simulink model "Aloe_E_Cell_Project_2016"  (R2016b)
settings: Solver=VariableStepAuto  StartTime=0.0  StopTime=0.14  RelTol=1e-3
undefined symbols (not defined in the file): D1, Delta
libraries: powerlib x218, powerlib_meascontrol x6, simulink x2
(part 1 of 2)
settings Model: Creator=mdeat  LastModifiedBy=mdeat
settings DataIOCC: ReturnWorkspaceOutputs=on
settings SFSimCC: SimUseLocalCustomCode=on
settings RTWCC: RTWUseLocalCustomCode=on

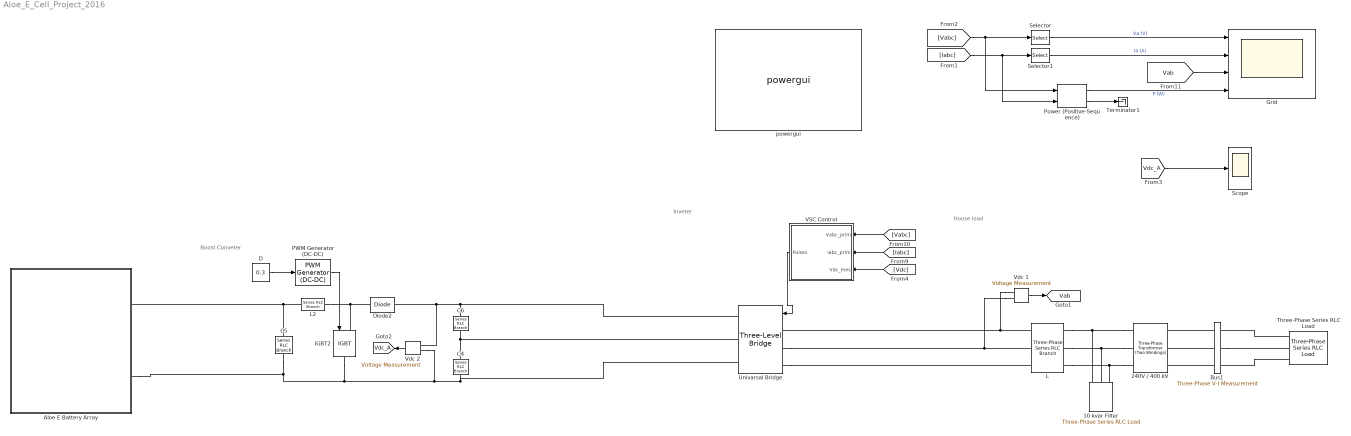
== system Aloe_E_Cell_Project_2016 ==
  note: Boost Conveter
  note: House load
  note: Inveter
  10 kvar Filter : powerlib/Elements/Three-Phase Series RLC Load  LConnTagsString=A|B|C  Configuration=Y (grounded)  NominalVoltage=240  Vabc=[1e3 1e3 1e3]  Vabcp=[1e3 1e3 1e3]  NominalFrequency=50  UnbalancedPower=off  ActivePower=100  InductivePower=0  CapacitivePower=10e3  Pabc=[10e3 9e3 11e3]  QLabc=[100 90 110]  QCabc=[100 90 110]  Pabcp=[10e3 9e3 11e3]  QLabcp=[100 90 110]  QCabcp=[100 90 110]  Measurements=None  LoadType=constant Z
  240V / 400 kV : powerlib/Elements/Three-Phase Transformer (Two Windings)  Winding1Connection=Yg  Winding2Connection=Delta (D1)  CoreType=Three single-phase transformers  SetSaturation=off  Hysteresis=off  DataFile='hysteresis'  SetInitialFlux=off  Measurements=None  UNITS=pu  NominalPower=[100 , 50 ]  Winding1=[ 400 , 0.001 , 0.03 ]  Winding2=[ 260 , 0.001 , 0.03 ]  Rm=500  Lm=500  L0=0.5  Saturation=[ 0,0 ; 0.0024,1.2 ; 1.0,1.52 ]  InitialFluxes=[ 0.8 , -0.8 , 0.7 ]  BreakLoop=off  DiscreteSolver=Trapezoidal iterative  DataType=off  TransfoNumber=0
  Aloe E Battery Array : Subsystem
      mask Display: image('$imagefile'); % Use "Edit Image" on toolstrip to change.
  Bus1 : powerlib/Measurements/Three-Phase V-I Measurement  VoltageMeasurement=phase-to-ground  SetLabelV=on  LabelV=Vabc  Vpu=off  VpuLL=off  CurrentMeasurement=yes  SetLabelI=on  LabelI=Iabc  Ipu=off  Pbase=100e6  Vbase=500e3  OutputType=Magnitude  PhasorSimulation=off  PSBequivalent=0
  C4 : powerlib/Elements/Series RLC Branch  LConnTagsString=__new0  RConnTagsString=__new0  BranchType=C  Resistance=1.0  Inductance=1.0  SetiL0=off  InitialCurrent=0  Capacitance=2e-4  Setx0=off  InitialVoltage=0  Measurements=None
  C5 : powerlib/Elements/Series RLC Branch  LConnTagsString=__new0  RConnTagsString=__new0  BranchType=C  Resistance=1.0  Inductance=1.0  SetiL0=off  InitialCurrent=0  Capacitance=100e-6  Setx0=off  InitialVoltage=0  Measurements=Branch voltage
  C6 : powerlib/Elements/Series RLC Branch  LConnTagsString=__new0  RConnTagsString=__new0  BranchType=C  Resistance=1.0  Inductance=1.0  SetiL0=off  InitialCurrent=0  Capacitance=12e-03  Setx0=off  InitialVoltage=0  Measurements=None
  D : Constant  Value=0.3
  Diode2 : powerlib/Power Electronics/Diode  Ron=1e-4  Lon=0  Vf=0  IC=0  UseSnubber=off  Rs=inf  Cs=inf  Measurements=off
  Grid : Scope  NumInputPorts=4
  IGBT2 : powerlib/Power Electronics/IGBT  Ron=0.001  Lon=0  Vf=0  Tf=0  Tt=0  IC=0  Rs=1e5  Cs=inf  Measurements=off
  L : powerlib/Elements/Three-Phase Series RLC Branch  LConnTagsString=A|B|C  RConnTagsString=A|B|C  BranchType=RL  Resistance=500e-6*377/50/2  Inductance=500e-6/2  Capacitance=inf  Measurements=None
  L2 : powerlib/Elements/Series RLC Branch  LConnTagsString=__new0  RConnTagsString=__new0  BranchType=RL  Resistance=0.005  Inductance=5e-3  SetiL0=off  InitialCurrent=0  Capacitance=1e-6  Setx0=off  InitialVoltage=0  Measurements=None
  PWM Generator (DC-DC) : powerlib_meascontrol/Pulse & Signal Generators/PWM Generator (DC-DC)  Fsw=20e3  Ts=0
  Power (Positive-Sequence) : powerlib_meascontrol/Measurements/Power (Positive-Sequence)  Freq=60  Vinit=[0, 0]  Iinit=[0, 0]  Ts=0.0001
  Scope : Scope
  Selector : Selector  InputPortWidth=3  IndexOptions=Index vector (dialog)  Indices=[1]  OutputSizes=1
  Selector1 : Selector  InputPortWidth=3  IndexOptions=Index vector (dialog)  Indices=[1]  OutputSizes=1
  Terminator1 : Terminator
  Three-Phase Series RLC Load : powerlib/Elements/Three-Phase Series RLC Load  LConnTagsString=A|B|C  Configuration=Y (grounded)  NominalVoltage=400  Vabc=[1e3 1e3 1e3]  Vabcp=[1e3 1e3 1e3]  NominalFrequency=50  UnbalancedPower=off  ActivePower=1000  InductivePower=0  CapacitivePower=100  Pabc=[10e3 9e3 11e3]  QLabc=[100 90 110]  QCabc=[100 90 110]  Pabcp=[10e3 9e3 11e3]  QLabcp=[100 90 110]  QCabcp=[100 90 110]  Measurements=None  LoadType=constant Z
  Univarsal Bridge : powerlib/Power Electronics/Three-Level Bridge  Arms=3  SnubberResistance=1e6  SbubberCapacitance=inf  Device=IGBT / Diodes  Ron=0.2e-3  ForwardVoltages="[  0  0 ]"  Measurements=None
  VSC Control : Subsystem  mask(VSC Main Controller){nom=[ 1000  50 ], Vnom=[ 2000 260 ], Vnom_dc=220, RLxfo=[0.002  0.06 ], RLchoke=[2e-3  250e-6  ], K_VDCreg=[7  800], K_Ireg=[0.3 20], Ts=0.0001}
      mask prompts: nom "Nominal power and frequency [ Pnom(VA)  Fnom(Hz) ]:"; Vnom "Nominal primary and secondary voltages (Vrms LL) [ Vnom_prim   Vnom_sec ]:"; Vnom_dc "Nominal DC bus voltage (V):"; RLxfo "Total transformer leakage impedance (pu/Pnom) [ Rxfo  Lxf ]"; RLchoke "Choke impedance [ R(ohm) L(H) ]"; K_VDCreg "VDC regultator gains [ Kp  Ki ]:"; K_Ireg "Current regulator gains [ Kp  Ki ]:"; Ts "Sample time"
      mask init:
      | Pnom=nom(1);
      | Fnom=nom(2);
      | Vnom_prim=Vnom(1);
      | Vnom_sec=Vnom(2);
      | Zbase=Vnom_sec^2/Pnom;
      | Rtot_pu=RLxfo(1) + RLchoke(1)/Zbase;
      | Ltot_pu=RLxfo(2) + RLchoke(2)/(Zbase/(2*pi*Fnom));
      | Kp_VDCreg=K_VDCreg(1);
      | Ki_VDCreg=K_VDCreg(2);
      | Kp_Ireg=K_Ireg(1);
      | Ki_Ireg=K_Ireg(2);
      | Vdc_ref=Vnom_dc;
      | % Used to determine initial value of Boost Control (MPPT)
      | assignin('base','Vdc_ref_Inv',Vdc_ref);
  Vdc 1 : powerlib/Measurements/Voltage Measurement  Tag=PoWeRsYsTeMmEaSuReMeNt  PhasorSimulation=off  OutputType=Magnitude  PSBequivalent=0
  Vdc 2 : powerlib/Measurements/Voltage Measurement  Tag=PoWeRsYsTeMmEaSuReMeNt  PhasorSimulation=off  OutputType=Magnitude  PSBequivalent=0
  powergui : powerlib/powergui  Priority=1  SimulationMode=Discrete  SampleTime=1e-5  frequency=60  Iterations=50  frequencyindice=0  Pbase=100e6  ErrMax=1e-4  UnitsV=kV  UnitsW=MW  buscounter=0  FunctionMessages=off  echomessages=off  EnableUseOfTLC=off  CurrentSourceSwitches=off  DisableSnubberDevices=off  DisableRonSwitches=off  DisableVfSwitches=off  DisplayEquations=off  AutomaticDiscreteSolvers=off  SolverType=Tustin/Backward Euler (TBE)  Interpol=off  ExternalGateDelay=off  methode=off  Ts=100  x0status=blocks  SPID=on  SwTol=0  HookPort=off  NonlinearTolerance=1e-4  nMaxIteration=100  ContinueOnMaxIteration=off  RestoreLinks=warning  ResistiveCurrentMeasurement=off  Frange=[0:2:500]  Ylog=off  Xlog=on  ShowGrid=off  save=off  variable=ZData  structure=0  ZoomFFT=off  StartTime=0.0  cycles=1  DisplayStyle=1  fundamental=60  FreqAxis=off  MaxFrequency=1000  frequencyindicesteady=1  RmsSteady=1  display=off
  tag scope: Vab=global, Vdc_A=global
  wires:
  Selector/1 -> Grid/1  "Va (V)"
  [Vab] -> Grid/3
  Selector1/1 -> Grid/2  "Ia (A)"
  [Vdc_A] -> Scope/1
  Power (Positive-Sequence)/1 -> Grid/4  "P (W)"
  Vdc 2/1 -> [Vdc_A]
  PWM Generator (DC-DC)/1 -> IGBT2/1
  D/1 -> PWM Generator (DC-DC)/1
  VSC Control/1(Pulses) -> Univarsal Bridge/1
  [Vabc] -> VSC Control/1(Vabc_prim)
  [Vdc] -> VSC Control/3(Vdc_mes)
  [Iabc] -> VSC Control/2(Iabc_prim)
  [Vabc] -> Power (Positive-Sequence)/1, Selector/1
  Power (Positive-Sequence)/2 -> Terminator1/1
  [Iabc] -> Power (Positive-Sequence)/2, Selector1/1
  Vdc 1/1 -> [Vab]
  connections:
  C5/LConn1 -- L2/LConn1 -- Aloe E Battery Array/RConn1
  Vdc 2/LConn2 -- Univarsal Bridge/RConn3 -- C4/RConn1 -- IGBT2/RConn1 -- C5/RConn1 -- Aloe E Battery Array/RConn2
  Diode2/RConn1 -- Univarsal Bridge/RConn1 -- C6/LConn1 -- Vdc 2/LConn1
  L2/RConn1 -- Diode2/LConn1 -- IGBT2/LConn1
  Vdc 1/LConn1 -- Univarsal Bridge/LConn1 -- L/LConn1
  240V / 400 kV/RConn3 -- L/RConn3 -- 10 kvar Filter/LConn3
  Vdc 1/LConn2 -- Univarsal Bridge/LConn2 -- L/LConn2
  240V / 400 kV/RConn1 -- L/RConn1 -- 10 kvar Filter/LConn1
  240V / 400 kV/RConn2 -- L/RConn2 -- 10 kvar Filter/LConn2
  Bus1/LConn3 -- 240V / 400 kV/LConn3
  Three-Phase Series RLC Load/LConn1 -- Bus1/RConn1
  Three-Phase Series RLC Load/LConn3 -- Bus1/RConn3
  Bus1/RConn2 -- Three-Phase Series RLC Load/LConn2
  Bus1/LConn2 -- 240V / 400 kV/LConn2
  Bus1/LConn1 -- 240V / 400 kV/LConn1
  Univarsal Bridge/LConn3 -- L/LConn3
  C4/LConn1 -- Univarsal Bridge/RConn2 -- C6/RConn1

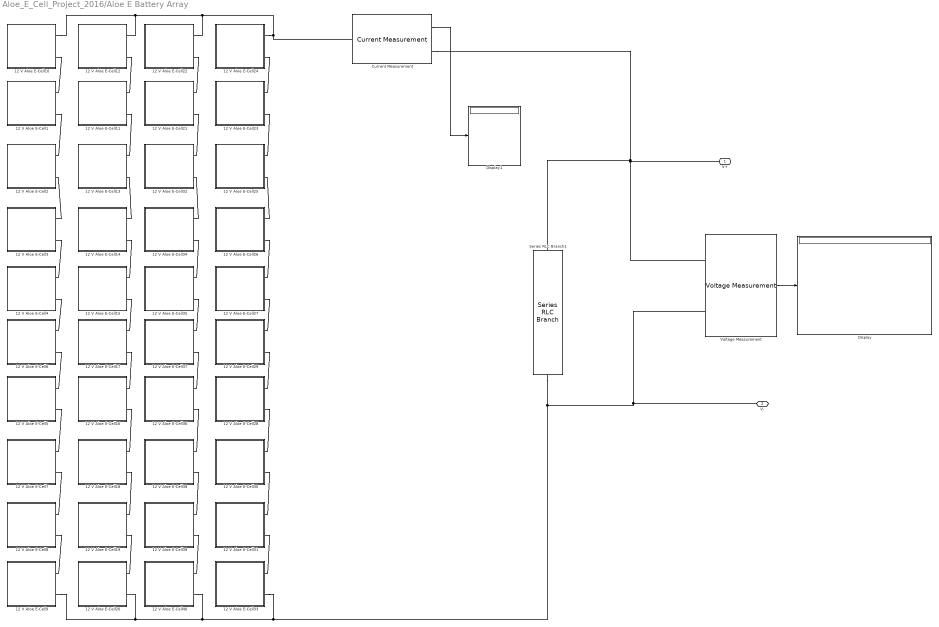
== system Aloe_E_Cell_Project_2016/Aloe E Battery Array ==
  12 V Aloe E-Cell1 : Subsystem
      mask Display: image('$imagefile'); % Use "Edit Image" on toolstrip to change.
  12 V Aloe E-Cell10 : Subsystem
      mask Display: image('$imagefile'); % Use "Edit Image" on toolstrip to change.
  12 V Aloe E-Cell11 : Subsystem
      mask Display: image('$imagefile'); % Use "Edit Image" on toolstrip to change.
  12 V Aloe E-Cell12 : Subsystem
      mask Display: image('$imagefile'); % Use "Edit Image" on toolstrip to change.
  12 V Aloe E-Cell13 : Subsystem
      mask Display: image('$imagefile'); % Use "Edit Image" on toolstrip to change.
  12 V Aloe E-Cell14 : Subsystem
      mask Display: image('$imagefile'); % Use "Edit Image" on toolstrip to change.
  12 V Aloe E-Cell15 : Subsystem
      mask Display: image('$imagefile'); % Use "Edit Image" on toolstrip to change.
  12 V Aloe E-Cell16 : Subsystem
      mask Display: image('$imagefile'); % Use "Edit Image" on toolstrip to change.
  12 V Aloe E-Cell17 : Subsystem
      mask Display: image('$imagefile'); % Use "Edit Image" on toolstrip to change.
  12 V Aloe E-Cell18 : Subsystem
      mask Display: image('$imagefile'); % Use "Edit Image" on toolstrip to change.
  12 V Aloe E-Cell19 : Subsystem
      mask Display: image('$imagefile'); % Use "Edit Image" on toolstrip to change.
  12 V Aloe E-Cell2 : Subsystem
      mask Display: image('$imagefile'); % Use "Edit Image" on toolstrip to change.
  12 V Aloe E-Cell20 : Subsystem
      mask Display: image('$imagefile'); % Use "Edit Image" on toolstrip to change.
  12 V Aloe E-Cell21 : Subsystem
      mask Display: image('$imagefile'); % Use "Edit Image" on toolstrip to change.
  12 V Aloe E-Cell22 : Subsystem
      mask Display: image('$imagefile'); % Use "Edit Image" on toolstrip to change.
  12 V Aloe E-Cell23 : Subsystem
      mask Display: image('$imagefile'); % Use "Edit Image" on toolstrip to change.
  12 V Aloe E-Cell24 : Subsystem
      mask Display: image('$imagefile'); % Use "Edit Image" on toolstrip to change.
  12 V Aloe E-Cell25 : Subsystem
      mask Display: image('$imagefile'); % Use "Edit Image" on toolstrip to change.
  12 V Aloe E-Cell26 : Subsystem
      mask Display: image('$imagefile'); % Use "Edit Image" on toolstrip to change.
  12 V Aloe E-Cell27 : Subsystem
      mask Display: image('$imagefile'); % Use "Edit Image" on toolstrip to change.
  12 V Aloe E-Cell28 : Subsystem
      mask Display: image('$imagefile'); % Use "Edit Image" on toolstrip to change.
  12 V Aloe E-Cell29 : Subsystem
      mask Display: image('$imagefile'); % Use "Edit Image" on toolstrip to change.
  12 V Aloe E-Cell3 : Subsystem
      mask Display: image('$imagefile'); % Use "Edit Image" on toolstrip to change.
  12 V Aloe E-Cell30 : Subsystem
      mask Display: image('$imagefile'); % Use "Edit Image" on toolstrip to change.
  12 V Aloe E-Cell31 : Subsystem
      mask Display: image('$imagefile'); % Use "Edit Image" on toolstrip to change.
  12 V Aloe E-Cell32 : Subsystem
      mask Display: image('$imagefile'); % Use "Edit Image" on toolstrip to change.
  12 V Aloe E-Cell33 : Subsystem
      mask Display: image('$imagefile'); % Use "Edit Image" on toolstrip to change.
  12 V Aloe E-Cell34 : Subsystem
      mask Display: image('$imagefile'); % Use "Edit Image" on toolstrip to change.
  12 V Aloe E-Cell35 : Subsystem
      mask Display: image('$imagefile'); % Use "Edit Image" on toolstrip to change.
  12 V Aloe E-Cell36 : Subsystem
      mask Display: image('$imagefile'); % Use "Edit Image" on toolstrip to change.
  12 V Aloe E-Cell37 : Subsystem
      mask Display: image('$imagefile'); % Use "Edit Image" on toolstrip to change.
  12 V Aloe E-Cell38 : Subsystem
      mask Display: image('$imagefile'); % Use "Edit Image" on toolstrip to change.
  12 V Aloe E-Cell39 : Subsystem
      mask Display: image('$imagefile'); % Use "Edit Image" on toolstrip to change.
  12 V Aloe E-Cell4 : Subsystem
      mask Display: image('$imagefile'); % Use "Edit Image" on toolstrip to change.
  12 V Aloe E-Cell40 : Subsystem
      mask Display: image('$imagefile'); % Use "Edit Image" on toolstrip to change.
  12 V Aloe E-Cell5 : Subsystem
      mask Display: image('$imagefile'); % Use "Edit Image" on toolstrip to change.
  12 V Aloe E-Cell6 : Subsystem
      mask Display: image('$imagefile'); % Use "Edit Image" on toolstrip to change.
  12 V Aloe E-Cell7 : Subsystem
      mask Display: image('$imagefile'); % Use "Edit Image" on toolstrip to change.
  12 V Aloe E-Cell8 : Subsystem
      mask Display: image('$imagefile'); % Use "Edit Image" on toolstrip to change.
  12 V Aloe E-Cell9 : Subsystem
      mask Display: image('$imagefile'); % Use "Edit Image" on toolstrip to change.
  Current Measurement : powerlib/Measurements/Current Measurement  PhasorSimulation=off  OutputType=Complex  PSBequivalent=0
  Display : Display
  Display1 : Display
      settings: Decimation=3
  Series RLC Branch1 : powerlib/Elements/Series RLC Branch  LConnTagsString=__new0  RConnTagsString=__new0  BranchType=R  Resistance=75  Inductance=1e-3  SetiL0=off  InitialCurrent=0  Capacitance=1e-3  Setx0=off  InitialVoltage=0  Measurements=None
  Voltage Measurement : powerlib/Measurements/Voltage Measurement  PhasorSimulation=off  OutputType=Complex  PSBequivalent=0
  V+ : PMIOPort  Side=Right
  V- : PMIOPort  Port=2  Side=Right
  wires:
  Current Measurement/1 -> Display1/1
  Voltage Measurement/1 -> Display/1
  connections:
  12 V Aloe E-Cell3/RConn1 -- 12 V Aloe E-Cell2/RConn2
  12 V Aloe E-Cell29/RConn2 -- 12 V Aloe E-Cell28/RConn1
  12 V Aloe E-Cell18/RConn2 -- 12 V Aloe E-Cell19/RConn1
  Voltage Measurement/LConn2 -- V-/RConn1 -- 12 V Aloe E-Cell33/RConn2 -- 12 V Aloe E-Cell20/RConn2 -- 12 V Aloe E-Cell9/RConn2 -- 12 V Aloe E-Cell40/RConn2 -- Series RLC Branch1/RConn1
  Series RLC Branch1/LConn1 -- Voltage Measurement/LConn1 -- V+/RConn1 -- Current Measurement/RConn1
  12 V Aloe E-Cell10/RConn1 -- Current Measurement/LConn1 -- 12 V Aloe E-Cell24/RConn1 -- 12 V Aloe E-Cell22/RConn1 -- 12 V Aloe E-Cell12/RConn1
  12 V Aloe E-Cell14/RConn2 -- 12 V Aloe E-Cell15/RConn1
  12 V Aloe E-Cell12/RConn2 -- 12 V Aloe E-Cell11/RConn1
  12 V Aloe E-Cell7/RConn2 -- 12 V Aloe E-Cell8/RConn1
  12 V Aloe E-Cell36/RConn2 -- 12 V Aloe E-Cell38/RConn1
  12 V Aloe E-Cell28/RConn2 -- 12 V Aloe E-Cell30/RConn1
  12 V Aloe E-Cell35/RConn2 -- 12 V Aloe E-Cell37/RConn1
  12 V Aloe E-Cell26/RConn1 -- 12 V Aloe E-Cell25/RConn2
  12 V Aloe E-Cell3/RConn2 -- 12 V Aloe E-Cell4/RConn1
  12 V Aloe E-Cell19/RConn2 -- 12 V Aloe E-Cell20/RConn1
  12 V Aloe E-Cell6/RConn2 -- 12 V Aloe E-Cell5/RConn1
  12 V Aloe E-Cell14/RConn1 -- 12 V Aloe E-Cell13/RConn2
  12 V Aloe E-Cell24/RConn2 -- 12 V Aloe E-Cell23/RConn1
  12 V Aloe E-Cell11/RConn2 -- 12 V Aloe E-Cell13/RConn1
  12 V Aloe E-Cell15/RConn2 -- 12 V Aloe E-Cell17/RConn1
  12 V Aloe E-Cell16/RConn2 -- 12 V Aloe E-Cell18/RConn1
  12 V Aloe E-Cell23/RConn2 -- 12 V Aloe E-Cell25/RConn1
  12 V Aloe E-Cell38/RConn2 -- 12 V Aloe E-Cell39/RConn1
  12 V Aloe E-Cell17/RConn2 -- 12 V Aloe E-Cell16/RConn1
  12 V Aloe E-Cell26/RConn2 -- 12 V Aloe E-Cell27/RConn1
  12 V Aloe E-Cell30/RConn2 -- 12 V Aloe E-Cell31/RConn1
  12 V Aloe E-Cell27/RConn2 -- 12 V Aloe E-Cell29/RConn1
  12 V Aloe E-Cell34/RConn1 -- 12 V Aloe E-Cell32/RConn2
  12 V Aloe E-Cell1/RConn2 -- 12 V Aloe E-Cell2/RConn1
  12 V Aloe E-Cell4/RConn2 -- 12 V Aloe E-Cell6/RConn1
  12 V Aloe E-Cell5/RConn2 -- 12 V Aloe E-Cell7/RConn1
  12 V Aloe E-Cell8/RConn2 -- 12 V Aloe E-Cell9/RConn1
  12 V Aloe E-Cell10/RConn2 -- 12 V Aloe E-Cell1/RConn1
  12 V Aloe E-Cell34/RConn2 -- 12 V Aloe E-Cell35/RConn1
  12 V Aloe E-Cell39/RConn2 -- 12 V Aloe E-Cell40/RConn1
  12 V Aloe E-Cell21/RConn2 -- 12 V Aloe E-Cell32/RConn1
  12 V Aloe E-Cell22/RConn2 -- 12 V Aloe E-Cell21/RConn1
  12 V Aloe E-Cell37/RConn2 -- 12 V Aloe E-Cell36/RConn1
  12 V Aloe E-Cell31/RConn2 -- 12 V Aloe E-Cell33/RConn1

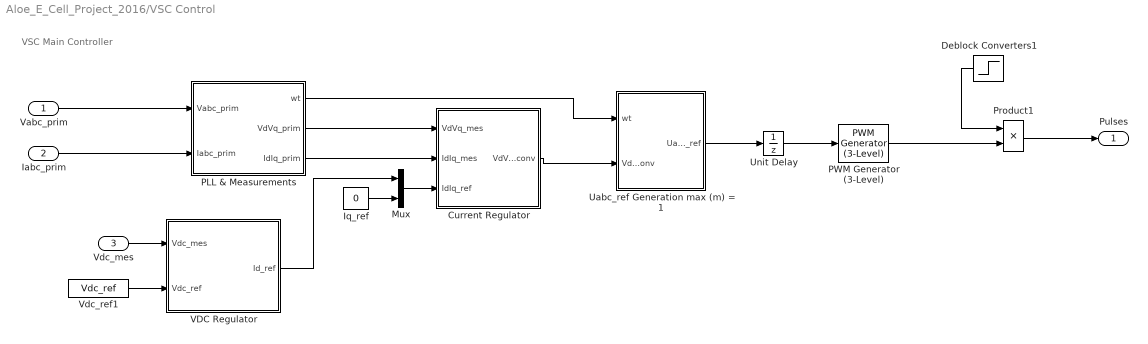
== system Aloe_E_Cell_Project_2016/VSC Control ==
  note: VSC Main Controller
  Vabc_prim : Inport  PortDimensions=3
  Iabc_prim : Inport  Port=2  PortDimensions=3
  Vdc_mes : Inport  Port=3  PortDimensions=1
  Current Regulator : Subsystem
  Deblock Converters1 : Step  Time=0.05  SampleTime=0
  Iq_ref : Constant  Value=0
  Mux : Mux  Inputs=2
  PLL & Measurements : Subsystem
  PWM Generator (3-Level) : powerlib_meascontrol/Pulse & Signal Generators/PWM Generator (3-Level)  ModulatorType=Three-phase bridge (12 pulses)  ModulatorMode=Unsynchronized  nF=27  Fc=33*60  ModulatingSignals=off  m=0.8  Freq=60  Phase=0  Ts=1e-6
  Product1 : Product  RndMeth=Zero
  Uabc_ref Generation max (m) = 1 : Subsystem
  Unit Delay : UnitDelay  SampleTime=0.0001  HasFrameUpgradeWarning=on
  VDC Regulator : Subsystem
  Vdc_ref1 : Constant  Value=Vdc_ref
  Pulses : Outport
  wires:
  VDC Regulator/1(Id_ref) -> Mux/1
  PLL & Measurements/1(wt) -> Uabc_ref Generation max (m) = 1/1(wt)
  Current Regulator/1(VdVq_conv) -> Uabc_ref Generation max (m) = 1/2(VdVq_conv)
  Iq_ref/1 -> Mux/2
  Mux/1 -> Current Regulator/3(IdIq_ref)
  PLL & Measurements/3(IdIq_prim) -> Current Regulator/2(IdIq_mes)
  PLL & Measurements/2(VdVq_prim) -> Current Regulator/1(VdVq_mes)
  Vdc_mes/1 -> VDC Regulator/1(Vdc_mes)
  Vabc_prim/1 -> PLL & Measurements/1(Vabc_prim)
  Iabc_prim/1 -> PLL & Measurements/2(Iabc_prim)
  Unit Delay/1 -> PWM Generator (3-Level)/1
  Uabc_ref Generation max (m) = 1/1(Uabc_ref) -> Unit Delay/1
  Vdc_ref1/1 -> VDC Regulator/2(Vdc_ref)
  Deblock Converters1/1 -> Product1/1
  Product1/1 -> Pulses/1
  PWM Generator (3-Level)/1 -> Product1/2

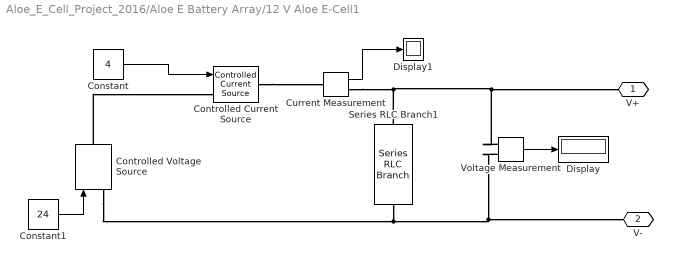
== system Aloe_E_Cell_Project_2016/Aloe E Battery Array/12 V Aloe E-Cell1 ==
  Constant : Constant  Value=4
  Constant1 : Constant  Value=24
  Controlled Current Source : powerlib/Electrical Sources/Controlled Current Source  Initialize=on  Source_Type=DC  Amplitude=1  Phase=0  Frequency=0  Measurements=None
  Controlled Voltage Source : powerlib/Electrical Sources/Controlled Voltage Source  Initialize=on  Source_Type=DC  Amplitude=1  Phase=0  Frequency=0  Measurements=Voltage
  Current Measurement : powerlib/Measurements/Current Measurement  PhasorSimulation=off  OutputType=Complex  PSBequivalent=0
  Display : Display
      settings: Decimation=3
  Display1 : Display
      settings: Decimation=3
  Series RLC Branch1 : powerlib/Elements/Series RLC Branch  LConnTagsString=__new0  RConnTagsString=__new0  BranchType=R  Resistance=6  Inductance=1e-3  SetiL0=off  InitialCurrent=0  Capacitance=1e-6  Setx0=off  InitialVoltage=0  Measurements=None
  Voltage Measurement : powerlib/Measurements/Voltage Measurement  PhasorSimulation=off  OutputType=Complex  PSBequivalent=0
  V+ : PMIOPort  Side=Right
  "V- " : PMIOPort  Port=2  Side=Right
  wires:
  Constant/1 -> Controlled Current Source/1
  Constant1/1 -> Controlled Voltage Source/1
  Current Measurement/1 -> Display1/1
  Voltage Measurement/1 -> Display/1
  connections:
  Series RLC Branch1/LConn1 -- Current Measurement/RConn1 -- Voltage Measurement/LConn1 -- V+/RConn1
  Controlled Voltage Source/RConn1 -- Controlled Current Source/LConn1
  Controlled Voltage Source/LConn1 -- Series RLC Branch1/RConn1 -- Voltage Measurement/LConn2 -- "V- "/RConn1
  Controlled Current Source/RConn1 -- Current Measurement/LConn1

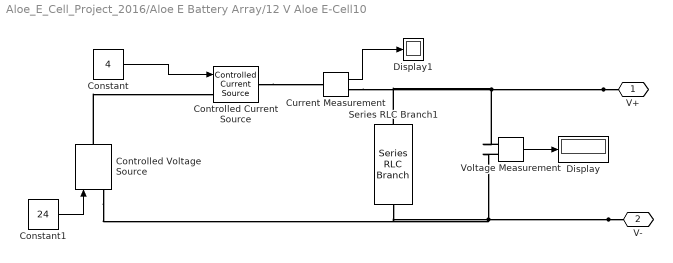
== system Aloe_E_Cell_Project_2016/Aloe E Battery Array/12 V Aloe E-Cell10 ==
  Constant : Constant  Value=4
  Constant1 : Constant  Value=24
  Controlled Current Source : powerlib/Electrical Sources/Controlled Current Source  Initialize=on  Source_Type=DC  Amplitude=1  Phase=0  Frequency=0  Measurements=None
  Controlled Voltage Source : powerlib/Electrical Sources/Controlled Voltage Source  Initialize=on  Source_Type=DC  Amplitude=1  Phase=0  Frequency=0  Measurements=Voltage
  Current Measurement : powerlib/Measurements/Current Measurement  PhasorSimulation=off  OutputType=Complex  PSBequivalent=0
  Display : Display
      settings: Decimation=3
  Display1 : Display
      settings: Decimation=3
  Series RLC Branch1 : powerlib/Elements/Series RLC Branch  LConnTagsString=__new0  RConnTagsString=__new0  BranchType=R  Resistance=6  Inductance=1e-3  SetiL0=off  InitialCurrent=0  Capacitance=1e-6  Setx0=off  InitialVoltage=0  Measurements=None
  Voltage Measurement : powerlib/Measurements/Voltage Measurement  PhasorSimulation=off  OutputType=Complex  PSBequivalent=0
  V+ : PMIOPort  Side=Right
  "V- " : PMIOPort  Port=2  Side=Right
  wires:
  Voltage Measurement/1 -> Display/1
  Current Measurement/1 -> Display1/1
  Constant1/1 -> Controlled Voltage Source/1
  Constant/1 -> Controlled Current Source/1
  connections:
  Controlled Current Source/RConn1 -- Current Measurement/LConn1
  "V- "/RConn1 -- Voltage Measurement/LConn2 -- Series RLC Branch1/RConn1 -- Controlled Voltage Source/LConn1
  Controlled Voltage Source/RConn1 -- Controlled Current Source/LConn1
  V+/RConn1 -- Voltage Measurement/LConn1 -- Current Measurement/RConn1 -- Series RLC Branch1/LConn1

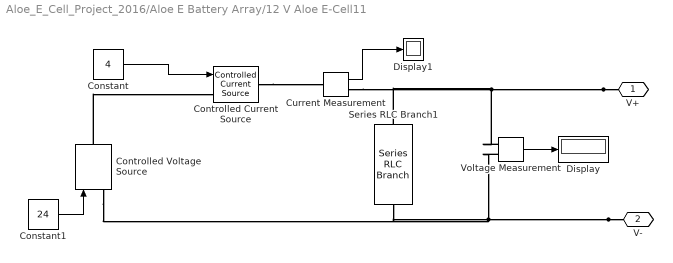
== system Aloe_E_Cell_Project_2016/Aloe E Battery Array/12 V Aloe E-Cell11 ==
  Constant : Constant  Value=4
  Constant1 : Constant  Value=24
  Controlled Current Source : powerlib/Electrical Sources/Controlled Current Source  Initialize=on  Source_Type=DC  Amplitude=1  Phase=0  Frequency=0  Measurements=None
  Controlled Voltage Source : powerlib/Electrical Sources/Controlled Voltage Source  Initialize=on  Source_Type=DC  Amplitude=1  Phase=0  Frequency=0  Measurements=Voltage
  Current Measurement : powerlib/Measurements/Current Measurement  PhasorSimulation=off  OutputType=Complex  PSBequivalent=0
  Display : Display
      settings: Decimation=3
  Display1 : Display
      settings: Decimation=3
  Series RLC Branch1 : powerlib/Elements/Series RLC Branch  LConnTagsString=__new0  RConnTagsString=__new0  BranchType=R  Resistance=6  Inductance=1e-3  SetiL0=off  InitialCurrent=0  Capacitance=1e-6  Setx0=off  InitialVoltage=0  Measurements=None
  Voltage Measurement : powerlib/Measurements/Voltage Measurement  PhasorSimulation=off  OutputType=Complex  PSBequivalent=0
  V+ : PMIOPort  Side=Right
  "V- " : PMIOPort  Port=2  Side=Right
  wires:
  Voltage Measurement/1 -> Display/1
  Current Measurement/1 -> Display1/1
  Constant1/1 -> Controlled Voltage Source/1
  Constant/1 -> Controlled Current Source/1
  connections:
  Controlled Current Source/RConn1 -- Current Measurement/LConn1
  "V- "/RConn1 -- Voltage Measurement/LConn2 -- Series RLC Branch1/RConn1 -- Controlled Voltage Source/LConn1
  Controlled Voltage Source/RConn1 -- Controlled Current Source/LConn1
  V+/RConn1 -- Voltage Measurement/LConn1 -- Current Measurement/RConn1 -- Series RLC Branch1/LConn1

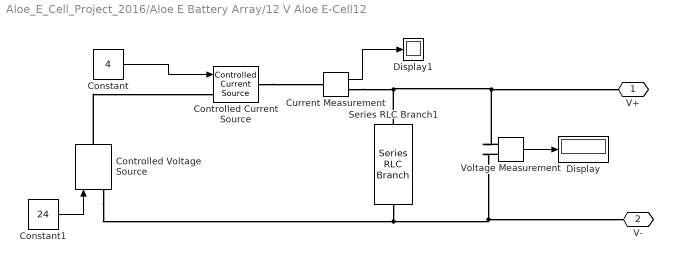
== system Aloe_E_Cell_Project_2016/Aloe E Battery Array/12 V Aloe E-Cell12 ==
  Constant : Constant  Value=4
  Constant1 : Constant  Value=24
  Controlled Current Source : powerlib/Electrical Sources/Controlled Current Source  Initialize=on  Source_Type=DC  Amplitude=1  Phase=0  Frequency=0  Measurements=None
  Controlled Voltage Source : powerlib/Electrical Sources/Controlled Voltage Source  Initialize=on  Source_Type=DC  Amplitude=1  Phase=0  Frequency=0  Measurements=Voltage
  Current Measurement : powerlib/Measurements/Current Measurement  PhasorSimulation=off  OutputType=Complex  PSBequivalent=0
  Display : Display
      settings: Decimation=3
  Display1 : Display
      settings: Decimation=3
  Series RLC Branch1 : powerlib/Elements/Series RLC Branch  LConnTagsString=__new0  RConnTagsString=__new0  BranchType=R  Resistance=6  Inductance=1e-3  SetiL0=off  InitialCurrent=0  Capacitance=1e-6  Setx0=off  InitialVoltage=0  Measurements=None
  Voltage Measurement : powerlib/Measurements/Voltage Measurement  PhasorSimulation=off  OutputType=Complex  PSBequivalent=0
  V+ : PMIOPort  Side=Right
  "V- " : PMIOPort  Port=2  Side=Right
  wires:
  Constant/1 -> Controlled Current Source/1
  Constant1/1 -> Controlled Voltage Source/1
  Current Measurement/1 -> Display1/1
  Voltage Measurement/1 -> Display/1
  connections:
  Series RLC Branch1/LConn1 -- Current Measurement/RConn1 -- Voltage Measurement/LConn1 -- V+/RConn1
  Controlled Voltage Source/RConn1 -- Controlled Current Source/LConn1
  Controlled Voltage Source/LConn1 -- Series RLC Branch1/RConn1 -- Voltage Measurement/LConn2 -- "V- "/RConn1
  Controlled Current Source/RConn1 -- Current Measurement/LConn1

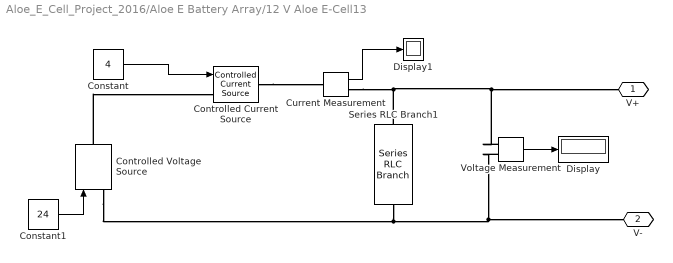
== system Aloe_E_Cell_Project_2016/Aloe E Battery Array/12 V Aloe E-Cell13 ==
  Constant : Constant  Value=4
  Constant1 : Constant  Value=24
  Controlled Current Source : powerlib/Electrical Sources/Controlled Current Source  Initialize=on  Source_Type=DC  Amplitude=1  Phase=0  Frequency=0  Measurements=None
  Controlled Voltage Source : powerlib/Electrical Sources/Controlled Voltage Source  Initialize=on  Source_Type=DC  Amplitude=1  Phase=0  Frequency=0  Measurements=Voltage
  Current Measurement : powerlib/Measurements/Current Measurement  PhasorSimulation=off  OutputType=Complex  PSBequivalent=0
  Display : Display
      settings: Decimation=3
  Display1 : Display
      settings: Decimation=3
  Series RLC Branch1 : powerlib/Elements/Series RLC Branch  LConnTagsString=__new0  RConnTagsString=__new0  BranchType=R  Resistance=6  Inductance=1e-3  SetiL0=off  InitialCurrent=0  Capacitance=1e-6  Setx0=off  InitialVoltage=0  Measurements=None
  Voltage Measurement : powerlib/Measurements/Voltage Measurement  PhasorSimulation=off  OutputType=Complex  PSBequivalent=0
  V+ : PMIOPort  Side=Right
  "V- " : PMIOPort  Port=2  Side=Right
  wires:
  Constant/1 -> Controlled Current Source/1
  Constant1/1 -> Controlled Voltage Source/1
  Current Measurement/1 -> Display1/1
  Voltage Measurement/1 -> Display/1
  connections:
  Series RLC Branch1/LConn1 -- Current Measurement/RConn1 -- Voltage Measurement/LConn1 -- V+/RConn1
  Controlled Voltage Source/RConn1 -- Controlled Current Source/LConn1
  Controlled Voltage Source/LConn1 -- Series RLC Branch1/RConn1 -- Voltage Measurement/LConn2 -- "V- "/RConn1
  Controlled Current Source/RConn1 -- Current Measurement/LConn1

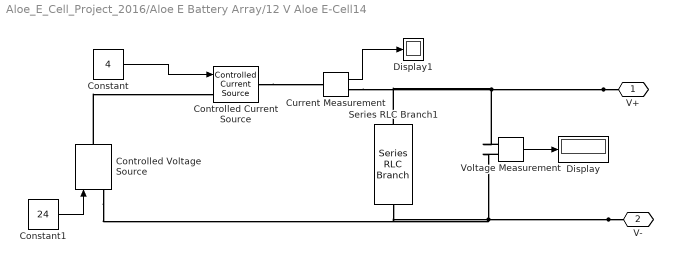
== system Aloe_E_Cell_Project_2016/Aloe E Battery Array/12 V Aloe E-Cell14 ==
  Constant : Constant  Value=4
  Constant1 : Constant  Value=24
  Controlled Current Source : powerlib/Electrical Sources/Controlled Current Source  Initialize=on  Source_Type=DC  Amplitude=1  Phase=0  Frequency=0  Measurements=None
  Controlled Voltage Source : powerlib/Electrical Sources/Controlled Voltage Source  Initialize=on  Source_Type=DC  Amplitude=1  Phase=0  Frequency=0  Measurements=Voltage
  Current Measurement : powerlib/Measurements/Current Measurement  PhasorSimulation=off  OutputType=Complex  PSBequivalent=0
  Display : Display
      settings: Decimation=3
  Display1 : Display
      settings: Decimation=3
  Series RLC Branch1 : powerlib/Elements/Series RLC Branch  LConnTagsString=__new0  RConnTagsString=__new0  BranchType=R  Resistance=6  Inductance=1e-3  SetiL0=off  InitialCurrent=0  Capacitance=1e-6  Setx0=off  InitialVoltage=0  Measurements=None
  Voltage Measurement : powerlib/Measurements/Voltage Measurement  PhasorSimulation=off  OutputType=Complex  PSBequivalent=0
  V+ : PMIOPort  Side=Right
  "V- " : PMIOPort  Port=2  Side=Right
  wires:
  Voltage Measurement/1 -> Display/1
  Current Measurement/1 -> Display1/1
  Constant1/1 -> Controlled Voltage Source/1
  Constant/1 -> Controlled Current Source/1
  connections:
  Controlled Current Source/RConn1 -- Current Measurement/LConn1
  "V- "/RConn1 -- Voltage Measurement/LConn2 -- Series RLC Branch1/RConn1 -- Controlled Voltage Source/LConn1
  Controlled Voltage Source/RConn1 -- Controlled Current Source/LConn1
  V+/RConn1 -- Voltage Measurement/LConn1 -- Current Measurement/RConn1 -- Series RLC Branch1/LConn1

== system Aloe_E_Cell_Project_2016/Aloe E Battery Array/12 V Aloe E-Cell15 ==
  Constant : Constant  Value=4
  Constant1 : Constant  Value=24
  Controlled Current Source : powerlib/Electrical Sources/Controlled Current Source  Initialize=on  Source_Type=DC  Amplitude=1  Phase=0  Frequency=0  Measurements=None
  Controlled Voltage Source : powerlib/Electrical Sources/Controlled Voltage Source  Initialize=on  Source_Type=DC  Amplitude=1  Phase=0  Frequency=0  Measurements=Voltage
  Current Measurement : powerlib/Measurements/Current Measurement  PhasorSimulation=off  OutputType=Complex  PSBequivalent=0
  Display : Display
      settings: Decimation=3
  Display1 : Display
      settings: Decimation=3
  Series RLC Branch1 : powerlib/Elements/Series RLC Branch  LConnTagsString=__new0  RConnTagsString=__new0  BranchType=R  Resistance=6  Inductance=1e-3  SetiL0=off  InitialCurrent=0  Capacitance=1e-6  Setx0=off  InitialVoltage=0  Measurements=None
  Voltage Measurement : powerlib/Measurements/Voltage Measurement  PhasorSimulation=off  OutputType=Complex  PSBequivalent=0
  V+ : PMIOPort  Side=Right
  "V- " : PMIOPort  Port=2  Side=Right
  wires:
  Constant/1 -> Controlled Current Source/1
  Constant1/1 -> Controlled Voltage Source/1
  Current Measurement/1 -> Display1/1
  Voltage Measurement/1 -> Display/1
  connections:
  Series RLC Branch1/LConn1 -- Current Measurement/RConn1 -- Voltage Measurement/LConn1 -- V+/RConn1
  Controlled Voltage Source/RConn1 -- Controlled Current Source/LConn1
  Controlled Voltage Source/LConn1 -- Series RLC Branch1/RConn1 -- Voltage Measurement/LConn2 -- "V- "/RConn1
  Controlled Current Source/RConn1 -- Current Measurement/LConn1

== system Aloe_E_Cell_Project_2016/Aloe E Battery Array/12 V Aloe E-Cell16 ==
  Constant : Constant  Value=4
  Constant1 : Constant  Value=24
  Controlled Current Source : powerlib/Electrical Sources/Controlled Current Source  Initialize=on  Source_Type=DC  Amplitude=1  Phase=0  Frequency=0  Measurements=None
  Controlled Voltage Source : powerlib/Electrical Sources/Controlled Voltage Source  Initialize=on  Source_Type=DC  Amplitude=1  Phase=0  Frequency=0  Measurements=Voltage
  Current Measurement : powerlib/Measurements/Current Measurement  PhasorSimulation=off  OutputType=Complex  PSBequivalent=0
  Display : Display
      settings: Decimation=3
  Display1 : Display
      settings: Decimation=3
  Series RLC Branch1 : powerlib/Elements/Series RLC Branch  LConnTagsString=__new0  RConnTagsString=__new0  BranchType=R  Resistance=6  Inductance=1e-3  SetiL0=off  InitialCurrent=0  Capacitance=1e-6  Setx0=off  InitialVoltage=0  Measurements=None
  Voltage Measurement : powerlib/Measurements/Voltage Measurement  PhasorSimulation=off  OutputType=Complex  PSBequivalent=0
  V+ : PMIOPort  Side=Right
  "V- " : PMIOPort  Port=2  Side=Right
  wires:
  Constant/1 -> Controlled Current Source/1
  Constant1/1 -> Controlled Voltage Source/1
  Current Measurement/1 -> Display1/1
  Voltage Measurement/1 -> Display/1
  connections:
  Series RLC Branch1/LConn1 -- Current Measurement/RConn1 -- Voltage Measurement/LConn1 -- V+/RConn1
  Controlled Voltage Source/RConn1 -- Controlled Current Source/LConn1
  Controlled Voltage Source/LConn1 -- Series RLC Branch1/RConn1 -- Voltage Measurement/LConn2 -- "V- "/RConn1
  Controlled Current Source/RConn1 -- Current Measurement/LConn1

== system Aloe_E_Cell_Project_2016/Aloe E Battery Array/12 V Aloe E-Cell17 ==
  Constant : Constant  Value=4
  Constant1 : Constant  Value=24
  Controlled Current Source : powerlib/Electrical Sources/Controlled Current Source  Initialize=on  Source_Type=DC  Amplitude=1  Phase=0  Frequency=0  Measurements=None
  Controlled Voltage Source : powerlib/Electrical Sources/Controlled Voltage Source  Initialize=on  Source_Type=DC  Amplitude=1  Phase=0  Frequency=0  Measurements=Voltage
  Current Measurement : powerlib/Measurements/Current Measurement  PhasorSimulation=off  OutputType=Complex  PSBequivalent=0
  Display : Display
      settings: Decimation=3
  Display1 : Display
      settings: Decimation=3
  Series RLC Branch1 : powerlib/Elements/Series RLC Branch  LConnTagsString=__new0  RConnTagsString=__new0  BranchType=R  Resistance=6  Inductance=1e-3  SetiL0=off  InitialCurrent=0  Capacitance=1e-6  Setx0=off  InitialVoltage=0  Measurements=None
  Voltage Measurement : powerlib/Measurements/Voltage Measurement  PhasorSimulation=off  OutputType=Complex  PSBequivalent=0
  V+ : PMIOPort  Side=Right
  "V- " : PMIOPort  Port=2  Side=Right
  wires:
  Voltage Measurement/1 -> Display/1
  Current Measurement/1 -> Display1/1
  Constant1/1 -> Controlled Voltage Source/1
  Constant/1 -> Controlled Current Source/1
  connections:
  Controlled Current Source/RConn1 -- Current Measurement/LConn1
  "V- "/RConn1 -- Voltage Measurement/LConn2 -- Series RLC Branch1/RConn1 -- Controlled Voltage Source/LConn1
  Controlled Voltage Source/RConn1 -- Controlled Current Source/LConn1
  V+/RConn1 -- Voltage Measurement/LConn1 -- Current Measurement/RConn1 -- Series RLC Branch1/LConn1

== system Aloe_E_Cell_Project_2016/Aloe E Battery Array/12 V Aloe E-Cell18 ==
  Constant : Constant  Value=4
  Constant1 : Constant  Value=24
  Controlled Current Source : powerlib/Electrical Sources/Controlled Current Source  Initialize=on  Source_Type=DC  Amplitude=1  Phase=0  Frequency=0  Measurements=None
  Controlled Voltage Source : powerlib/Electrical Sources/Controlled Voltage Source  Initialize=on  Source_Type=DC  Amplitude=1  Phase=0  Frequency=0  Measurements=Voltage
  Current Measurement : powerlib/Measurements/Current Measurement  PhasorSimulation=off  OutputType=Complex  PSBequivalent=0
  Display : Display
      settings: Decimation=3
  Display1 : Display
      settings: Decimation=3
  Series RLC Branch1 : powerlib/Elements/Series RLC Branch  LConnTagsString=__new0  RConnTagsString=__new0  BranchType=R  Resistance=6  Inductance=1e-3  SetiL0=off  InitialCurrent=0  Capacitance=1e-6  Setx0=off  InitialVoltage=0  Measurements=None
  Voltage Measurement : powerlib/Measurements/Voltage Measurement  PhasorSimulation=off  OutputType=Complex  PSBequivalent=0
  V+ : PMIOPort  Side=Right
  "V- " : PMIOPort  Port=2  Side=Right
  wires:
  Voltage Measurement/1 -> Display/1
  Current Measurement/1 -> Display1/1
  Constant1/1 -> Controlled Voltage Source/1
  Constant/1 -> Controlled Current Source/1
  connections:
  Controlled Current Source/RConn1 -- Current Measurement/LConn1
  "V- "/RConn1 -- Voltage Measurement/LConn2 -- Series RLC Branch1/RConn1 -- Controlled Voltage Source/LConn1
  Controlled Voltage Source/RConn1 -- Controlled Current Source/LConn1
  V+/RConn1 -- Voltage Measurement/LConn1 -- Current Measurement/RConn1 -- Series RLC Branch1/LConn1

== system Aloe_E_Cell_Project_2016/Aloe E Battery Array/12 V Aloe E-Cell19 ==
  Constant : Constant  Value=4
  Constant1 : Constant  Value=24
  Controlled Current Source : powerlib/Electrical Sources/Controlled Current Source  Initialize=on  Source_Type=DC  Amplitude=1  Phase=0  Frequency=0  Measurements=None
  Controlled Voltage Source : powerlib/Electrical Sources/Controlled Voltage Source  Initialize=on  Source_Type=DC  Amplitude=1  Phase=0  Frequency=0  Measurements=Voltage
  Current Measurement : powerlib/Measurements/Current Measurement  PhasorSimulation=off  OutputType=Complex  PSBequivalent=0
  Display : Display
      settings: Decimation=3
  Display1 : Display
      settings: Decimation=3
  Series RLC Branch1 : powerlib/Elements/Series RLC Branch  LConnTagsString=__new0  RConnTagsString=__new0  BranchType=R  Resistance=6  Inductance=1e-3  SetiL0=off  InitialCurrent=0  Capacitance=1e-6  Setx0=off  InitialVoltage=0  Measurements=None
  Voltage Measurement : powerlib/Measurements/Voltage Measurement  PhasorSimulation=off  OutputType=Complex  PSBequivalent=0
  V+ : PMIOPort  Side=Right
  "V- " : PMIOPort  Port=2  Side=Right
  wires:
  Constant/1 -> Controlled Current Source/1
  Constant1/1 -> Controlled Voltage Source/1
  Current Measurement/1 -> Display1/1
  Voltage Measurement/1 -> Display/1
  connections:
  Series RLC Branch1/LConn1 -- Current Measurement/RConn1 -- Voltage Measurement/LConn1 -- V+/RConn1
  Controlled Voltage Source/RConn1 -- Controlled Current Source/LConn1
  Controlled Voltage Source/LConn1 -- Series RLC Branch1/RConn1 -- Voltage Measurement/LConn2 -- "V- "/RConn1
  Controlled Current Source/RConn1 -- Current Measurement/LConn1

== system Aloe_E_Cell_Project_2016/Aloe E Battery Array/12 V Aloe E-Cell2 ==
  Constant : Constant  Value=4
  Constant1 : Constant  Value=24
  Controlled Current Source : powerlib/Electrical Sources/Controlled Current Source  Initialize=on  Source_Type=DC  Amplitude=1  Phase=0  Frequency=0  Measurements=None
  Controlled Voltage Source : powerlib/Electrical Sources/Controlled Voltage Source  Initialize=on  Source_Type=DC  Amplitude=1  Phase=0  Frequency=0  Measurements=Voltage
  Current Measurement : powerlib/Measurements/Current Measurement  PhasorSimulation=off  OutputType=Complex  PSBequivalent=0
  Display : Display
      settings: Decimation=3
  Display1 : Display
      settings: Decimation=3
  Series RLC Branch1 : powerlib/Elements/Series RLC Branch  LConnTagsString=__new0  RConnTagsString=__new0  BranchType=R  Resistance=6  Inductance=1e-3  SetiL0=off  InitialCurrent=0  Capacitance=1e-6  Setx0=off  InitialVoltage=0  Measurements=None
  Voltage Measurement : powerlib/Measurements/Voltage Measurement  PhasorSimulation=off  OutputType=Complex  PSBequivalent=0
  V+ : PMIOPort  Side=Right
  "V- " : PMIOPort  Port=2  Side=Right
  wires:
  Voltage Measurement/1 -> Display/1
  Current Measurement/1 -> Display1/1
  Constant1/1 -> Controlled Voltage Source/1
  Constant/1 -> Controlled Current Source/1
  connections:
  Controlled Current Source/RConn1 -- Current Measurement/LConn1
  "V- "/RConn1 -- Voltage Measurement/LConn2 -- Series RLC Branch1/RConn1 -- Controlled Voltage Source/LConn1
  Controlled Voltage Source/RConn1 -- Controlled Current Source/LConn1
  V+/RConn1 -- Voltage Measurement/LConn1 -- Current Measurement/RConn1 -- Series RLC Branch1/LConn1

== system Aloe_E_Cell_Project_2016/Aloe E Battery Array/12 V Aloe E-Cell20 ==
  Constant : Constant  Value=4
  Constant1 : Constant  Value=24
  Controlled Current Source : powerlib/Electrical Sources/Controlled Current Source  Initialize=on  Source_Type=DC  Amplitude=1  Phase=0  Frequency=0  Measurements=None
  Controlled Voltage Source : powerlib/Electrical Sources/Controlled Voltage Source  Initialize=on  Source_Type=DC  Amplitude=1  Phase=0  Frequency=0  Measurements=Voltage
  Current Measurement : powerlib/Measurements/Current Measurement  PhasorSimulation=off  OutputType=Complex  PSBequivalent=0
  Display : Display
      settings: Decimation=3
  Display1 : Display
      settings: Decimation=3
  Series RLC Branch1 : powerlib/Elements/Series RLC Branch  LConnTagsString=__new0  RConnTagsString=__new0  BranchType=R  Resistance=6  Inductance=1e-3  SetiL0=off  InitialCurrent=0  Capacitance=1e-6  Setx0=off  InitialVoltage=0  Measurements=None
  Voltage Measurement : powerlib/Measurements/Voltage Measurement  PhasorSimulation=off  OutputType=Complex  PSBequivalent=0
  V+ : PMIOPort  Side=Right
  "V- " : PMIOPort  Port=2  Side=Right
  wires:
  Voltage Measurement/1 -> Display/1
  Current Measurement/1 -> Display1/1
  Constant1/1 -> Controlled Voltage Source/1
  Constant/1 -> Controlled Current Source/1
  connections:
  Controlled Current Source/RConn1 -- Current Measurement/LConn1
  "V- "/RConn1 -- Voltage Measurement/LConn2 -- Series RLC Branch1/RConn1 -- Controlled Voltage Source/LConn1
  Controlled Voltage Source/RConn1 -- Controlled Current Source/LConn1
  V+/RConn1 -- Voltage Measurement/LConn1 -- Current Measurement/RConn1 -- Series RLC Branch1/LConn1

== system Aloe_E_Cell_Project_2016/Aloe E Battery Array/12 V Aloe E-Cell21 ==
  Constant : Constant  Value=4
  Constant1 : Constant  Value=24
  Controlled Current Source : powerlib/Electrical Sources/Controlled Current Source  Initialize=on  Source_Type=DC  Amplitude=1  Phase=0  Frequency=0  Measurements=None
  Controlled Voltage Source : powerlib/Electrical Sources/Controlled Voltage Source  Initialize=on  Source_Type=DC  Amplitude=1  Phase=0  Frequency=0  Measurements=Voltage
  Current Measurement : powerlib/Measurements/Current Measurement  PhasorSimulation=off  OutputType=Complex  PSBequivalent=0
  Display : Display
      settings: Decimation=3
  Display1 : Display
      settings: Decimation=3
  Series RLC Branch1 : powerlib/Elements/Series RLC Branch  LConnTagsString=__new0  RConnTagsString=__new0  BranchType=R  Resistance=6  Inductance=1e-3  SetiL0=off  InitialCurrent=0  Capacitance=1e-6  Setx0=off  InitialVoltage=0  Measurements=None
  Voltage Measurement : powerlib/Measurements/Voltage Measurement  PhasorSimulation=off  OutputType=Complex  PSBequivalent=0
  V+ : PMIOPort  Side=Right
  "V- " : PMIOPort  Port=2  Side=Right
  wires:
  Voltage Measurement/1 -> Display/1
  Current Measurement/1 -> Display1/1
  Constant1/1 -> Controlled Voltage Source/1
  Constant/1 -> Controlled Current Source/1
  connections:
  Controlled Current Source/RConn1 -- Current Measurement/LConn1
  "V- "/RConn1 -- Voltage Measurement/LConn2 -- Series RLC Branch1/RConn1 -- Controlled Voltage Source/LConn1
  Controlled Voltage Source/RConn1 -- Controlled Current Source/LConn1
  V+/RConn1 -- Voltage Measurement/LConn1 -- Current Measurement/RConn1 -- Series RLC Branch1/LConn1

== system Aloe_E_Cell_Project_2016/Aloe E Battery Array/12 V Aloe E-Cell22 ==
  Constant : Constant  Value=4
  Constant1 : Constant  Value=24
  Controlled Current Source : powerlib/Electrical Sources/Controlled Current Source  Initialize=on  Source_Type=DC  Amplitude=1  Phase=0  Frequency=0  Measurements=None
  Controlled Voltage Source : powerlib/Electrical Sources/Controlled Voltage Source  Initialize=on  Source_Type=DC  Amplitude=1  Phase=0  Frequency=0  Measurements=Voltage
  Current Measurement : powerlib/Measurements/Current Measurement  PhasorSimulation=off  OutputType=Complex  PSBequivalent=0
  Display : Display
      settings: Decimation=3
  Display1 : Display
      settings: Decimation=3
  Series RLC Branch1 : powerlib/Elements/Series RLC Branch  LConnTagsString=__new0  RConnTagsString=__new0  BranchType=R  Resistance=6  Inductance=1e-3  SetiL0=off  InitialCurrent=0  Capacitance=1e-6  Setx0=off  InitialVoltage=0  Measurements=None
  Voltage Measurement : powerlib/Measurements/Voltage Measurement  PhasorSimulation=off  OutputType=Complex  PSBequivalent=0
  V+ : PMIOPort  Side=Right
  "V- " : PMIOPort  Port=2  Side=Right
  wires:
  Constant/1 -> Controlled Current Source/1
  Constant1/1 -> Controlled Voltage Source/1
  Current Measurement/1 -> Display1/1
  Voltage Measurement/1 -> Display/1
  connections:
  Series RLC Branch1/LConn1 -- Current Measurement/RConn1 -- Voltage Measurement/LConn1 -- V+/RConn1
  Controlled Voltage Source/RConn1 -- Controlled Current Source/LConn1
  Controlled Voltage Source/LConn1 -- Series RLC Branch1/RConn1 -- Voltage Measurement/LConn2 -- "V- "/RConn1
  Controlled Current Source/RConn1 -- Current Measurement/LConn1

== system Aloe_E_Cell_Project_2016/Aloe E Battery Array/12 V Aloe E-Cell23 ==
  Constant : Constant  Value=4
  Constant1 : Constant  Value=24
  Controlled Current Source : powerlib/Electrical Sources/Controlled Current Source  Initialize=on  Source_Type=DC  Amplitude=1  Phase=0  Frequency=0  Measurements=None
  Controlled Voltage Source : powerlib/Electrical Sources/Controlled Voltage Source  Initialize=on  Source_Type=DC  Amplitude=1  Phase=0  Frequency=0  Measurements=Voltage
  Current Measurement : powerlib/Measurements/Current Measurement  PhasorSimulation=off  OutputType=Complex  PSBequivalent=0
  Display : Display
      settings: Decimation=3
  Display1 : Display
      settings: Decimation=3
  Series RLC Branch1 : powerlib/Elements/Series RLC Branch  LConnTagsString=__new0  RConnTagsString=__new0  BranchType=R  Resistance=6  Inductance=1e-3  SetiL0=off  InitialCurrent=0  Capacitance=1e-6  Setx0=off  InitialVoltage=0  Measurements=None
  Voltage Measurement : powerlib/Measurements/Voltage Measurement  PhasorSimulation=off  OutputType=Complex  PSBequivalent=0
  V+ : PMIOPort  Side=Right
  "V- " : PMIOPort  Port=2  Side=Right
  wires:
  Constant/1 -> Controlled Current Source/1
  Constant1/1 -> Controlled Voltage Source/1
  Current Measurement/1 -> Display1/1
  Voltage Measurement/1 -> Display/1
  connections:
  Series RLC Branch1/LConn1 -- Current Measurement/RConn1 -- Voltage Measurement/LConn1 -- V+/RConn1
  Controlled Voltage Source/RConn1 -- Controlled Current Source/LConn1
  Controlled Voltage Source/LConn1 -- Series RLC Branch1/RConn1 -- Voltage Measurement/LConn2 -- "V- "/RConn1
  Controlled Current Source/RConn1 -- Current Measurement/LConn1

== system Aloe_E_Cell_Project_2016/Aloe E Battery Array/12 V Aloe E-Cell24 ==
  Constant : Constant  Value=4
  Constant1 : Constant  Value=24
  Controlled Current Source : powerlib/Electrical Sources/Controlled Current Source  Initialize=on  Source_Type=DC  Amplitude=1  Phase=0  Frequency=0  Measurements=None
  Controlled Voltage Source : powerlib/Electrical Sources/Controlled Voltage Source  Initialize=on  Source_Type=DC  Amplitude=1  Phase=0  Frequency=0  Measurements=Voltage
  Current Measurement : powerlib/Measurements/Current Measurement  PhasorSimulation=off  OutputType=Complex  PSBequivalent=0
  Display : Display
      settings: Decimation=3
  Display1 : Display
      settings: Decimation=3
  Series RLC Branch1 : powerlib/Elements/Series RLC Branch  LConnTagsString=__new0  RConnTagsString=__new0  BranchType=R  Resistance=6  Inductance=1e-3  SetiL0=off  InitialCurrent=0  Capacitance=1e-6  Setx0=off  InitialVoltage=0  Measurements=None
  Voltage Measurement : powerlib/Measurements/Voltage Measurement  PhasorSimulation=off  OutputType=Complex  PSBequivalent=0
  V+ : PMIOPort  Side=Right
  "V- " : PMIOPort  Port=2  Side=Right
  wires:
  Voltage Measurement/1 -> Display/1
  Current Measurement/1 -> Display1/1
  Constant1/1 -> Controlled Voltage Source/1
  Constant/1 -> Controlled Current Source/1
  connections:
  Controlled Current Source/RConn1 -- Current Measurement/LConn1
  "V- "/RConn1 -- Voltage Measurement/LConn2 -- Series RLC Branch1/RConn1 -- Controlled Voltage Source/LConn1
  Controlled Voltage Source/RConn1 -- Controlled Current Source/LConn1
  V+/RConn1 -- Voltage Measurement/LConn1 -- Current Measurement/RConn1 -- Series RLC Branch1/LConn1

== system Aloe_E_Cell_Project_2016/Aloe E Battery Array/12 V Aloe E-Cell25 ==
  Constant : Constant  Value=4
  Constant1 : Constant  Value=24
  Controlled Current Source : powerlib/Electrical Sources/Controlled Current Source  Initialize=on  Source_Type=DC  Amplitude=1  Phase=0  Frequency=0  Measurements=None
  Controlled Voltage Source : powerlib/Electrical Sources/Controlled Voltage Source  Initialize=on  Source_Type=DC  Amplitude=1  Phase=0  Frequency=0  Measurements=Voltage
  Current Measurement : powerlib/Measurements/Current Measurement  PhasorSimulation=off  OutputType=Complex  PSBequivalent=0
  Display : Display
      settings: Decimation=3
  Display1 : Display
      settings: Decimation=3
  Series RLC Branch1 : powerlib/Elements/Series RLC Branch  LConnTagsString=__new0  RConnTagsString=__new0  BranchType=R  Resistance=6  Inductance=1e-3  SetiL0=off  InitialCurrent=0  Capacitance=1e-6  Setx0=off  InitialVoltage=0  Measurements=None
  Voltage Measurement : powerlib/Measurements/Voltage Measurement  PhasorSimulation=off  OutputType=Complex  PSBequivalent=0
  V+ : PMIOPort  Side=Right
  "V- " : PMIOPort  Port=2  Side=Right
  wires:
  Voltage Measurement/1 -> Display/1
  Current Measurement/1 -> Display1/1
  Constant1/1 -> Controlled Voltage Source/1
  Constant/1 -> Controlled Current Source/1
  connections:
  Controlled Current Source/RConn1 -- Current Measurement/LConn1
  "V- "/RConn1 -- Voltage Measurement/LConn2 -- Series RLC Branch1/RConn1 -- Controlled Voltage Source/LConn1
  Controlled Voltage Source/RConn1 -- Controlled Current Source/LConn1
  V+/RConn1 -- Voltage Measurement/LConn1 -- Current Measurement/RConn1 -- Series RLC Branch1/LConn1
